simulink model "truck_LQR"  (Simulink 9.1)
settings: Solver=ode4  StartTime=0.0  StopTime=23  FixedStep=0.001  RelTol=1e-3  EnableMultiTasking=on
libraries: Solver_SF x1, simulink x1
settings Model: Creator=CIDI_xuhao  LastModifiedBy=DELL
settings DataIOCC: SaveFormat=Dataset
settings DebuggingCC: UnderspecifiedInitializationDetection=Simplified  MergeDetectMultiDrivingBlocksExec=error
settings HardwareCC: ProdBitPerPointer=64  ProdBitPerSizeT=64  ProdBitPerPtrDiffT=64  ProdLargestAtomicFloat=Float  ProdIntDivRoundTo=Zero  ProdEndianess=LittleEndian  ProdWordSize=64  ProdHWDeviceType=Intel->x86-64 (Windows64)
settings ModelReferenceCC: PropagateSignalLabelsOutOfModel=on
settings GRTTargetCC: GeneratePreprocessorConditionals=Disable all  CombineOutputUpdateFcns=on  GRTInterface=off

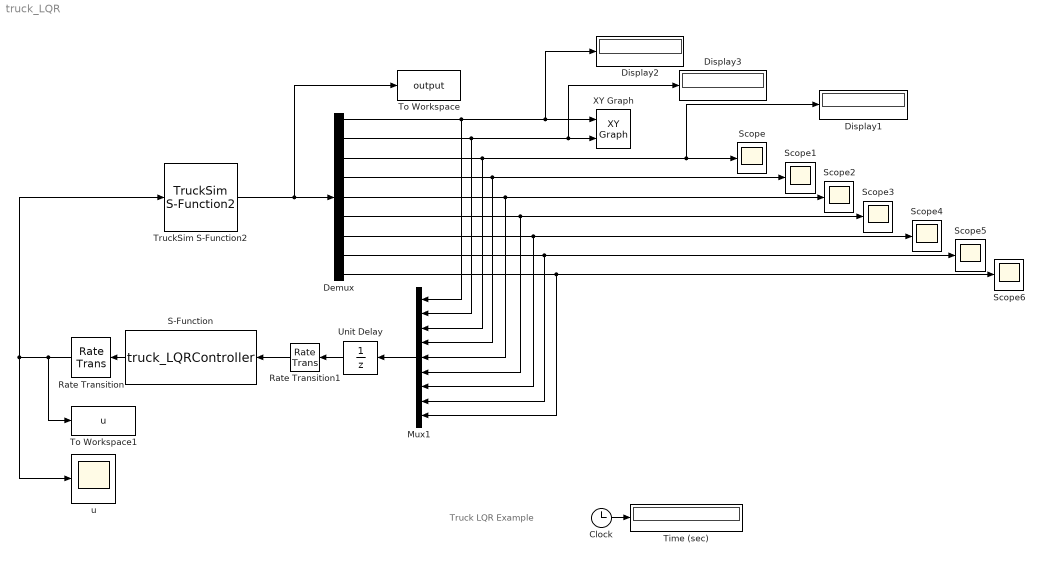
== system truck_LQR ==
  note: Truck LQR Example
  Clock : Clock
  Demux : Demux  Outputs=9
  Display1 : Display
  Display2 : Display
  Display3 : Display
  Mux1 : Mux  Inputs=9
  Rate Transition : RateTransition  OutPortSampleTime=0.001
  Rate Transition1 : RateTransition  OutPortSampleTime=0.01
  S-Function : S-Function  FunctionName=truck_LQRController  SFunctionDeploymentMode=off  EnableBusSupport=off
  Scope{,1..6} (7 alike) : Scope
  Time (sec) : Display
      settings: Format=bank  Decimation=100
  To Workspace : ToWorkspace  VariableName=output  SaveFormat=Timeseries  SampleTime=-1
  To Workspace1 : ToWorkspace  VariableName=u  SaveFormat=Timeseries  SampleTime=-1
  TruckSim S-Function2 : Solver_SF/TruckSim S-Function2  Priority=1  VehicleCode=s_ss__sss  SIMFILE=simfile.sim
      settings: AttributesFormatString=Vehicle Code: %<VehicleCode>
  Unit Delay : UnitDelay  SampleTime=-1
  XY Graph : simulink/Sinks/XY Graph  xmin=-110  xmax=150  ymin=-1  ymax=210  st=-1
  u : Scope
  wires:
  Unit Delay/1 -> Rate Transition1/1
  TruckSim S-Function2/1 -> To Workspace/1, Demux/1
  Demux/2 -> Mux1/2, Display3/1, XY Graph/2
  Demux/1 -> Mux1/1, Display2/1, XY Graph/1
  Demux/3 -> Mux1/3, Display1/1, Scope/1
  Demux/4 -> Mux1/4, Scope1/1
  Demux/5 -> Mux1/5, Scope2/1
  Mux1/1 -> Unit Delay/1
  S-Function/1 -> Rate Transition/1
  Clock/1 -> Time (sec)/1
  Demux/6 -> Mux1/6, Scope3/1
  Demux/7 -> Mux1/7, Scope4/1
  Demux/8 -> Mux1/8, Scope5/1
  Demux/9 -> Mux1/9, Scope6/1
  Rate Transition/1 -> To Workspace1/1, TruckSim S-Function2/1, u/1
  Rate Transition1/1 -> S-Function/1
